simulink model "cl2_2019"  (R2019b)
settings: Solver=VariableStepAuto  StartTime=0.0  StopTime=10.0  RelTol=1e-3
values from neighbouring files (symbols this model uses):
  A = [[0 0 1 0] ... (first row only)    [ClosedLoop.m]    (also in Inverted_pendulum.m; Realistic_model.m)
  B = [0 ... (first row only)    [ClosedLoop.m]    (also in Inverted_pendulum.m; Realistic_model.m)
  C = eye(n)    [ClosedLoop.m]    (also in Inverted_pendulum.m = [4.41/0.456, 0, 0, 0; Realistic_model.m = zeros(n,n); C(1,1) = 1; C(2,2) = 1)
  D = zeros(n,1)    [ClosedLoop.m]    (also in Inverted_pendulum.m = [0;0]; Realistic_model.m)
undefined symbols (not defined in the file or in its folder): K
settings Model: Creator=elina  LastModifiedBy=gebruiker

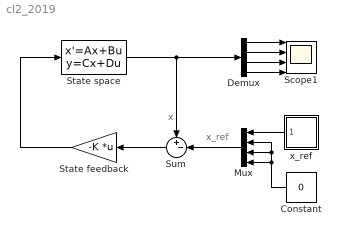
== system cl2_2019 ==
  note: x
  note: x_ref
  Constant : Constant  Value=0
  Demux : Demux
  Mux : Mux
  Scope1 : Scope  NumInputPorts=4
  State feedback : Gain  Gain=-K  Multiplication=Matrix(K*u)
  State space : StateSpace  A=A  B=B  C=C  D=D  InitialCondition=0
  Sum : Sum  Inputs=+-|
  x_ref : Subsystem
  wires:
  State space/1 -> Demux/1, Sum/1
  Demux/1 -> Scope1/1
  Demux/2 -> Scope1/2
  Demux/3 -> Scope1/3
  Demux/4 -> Scope1/4
  State feedback/1 -> State space/1
  Sum/1 -> State feedback/1
  Mux/1 -> Sum/2
  Constant/1 -> Mux/2, Mux/3, Mux/4
  x_ref/1(Out1) -> Mux/1

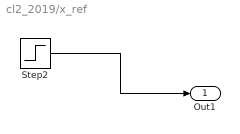
== system cl2_2019/x_ref ==
  Step2 : Step  After=0.04  SampleTime=0
  Out1 : Outport
  wires:
  Step2/1 -> Out1/1
